simulink model "Level0"  (R2021a)
settings: Solver=VariableStepAuto  StartTime=0.0  StopTime=10.0  RelTol=1e-3
settings Model: Creator=jpss8  LastModifiedBy=jpss8

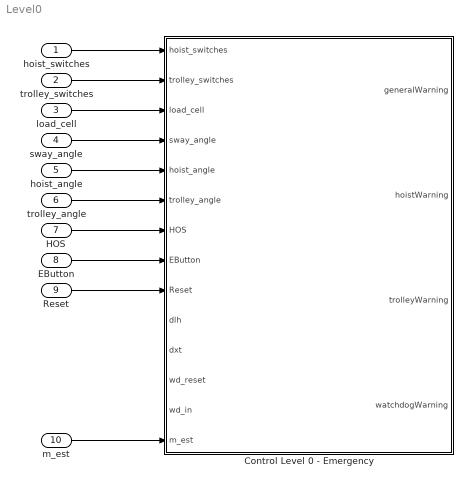
== system Level0 ==
  hoist_switches : Inport  PortDimensions=4
  trolley_switches : Inport  Port=2  PortDimensions=4
  load_cell : Inport  Port=3
  sway_angle : Inport  Port=4
  hoist_angle : Inport  Port=5
  trolley_angle : Inport  Port=6
  HOS : Inport  Port=7
  EButton : Inport  Port=8
  Reset : Inport  Port=9
  m_est : Inport  Port=10
  Control Level 0 - Emergency : Stateflow chart  TreatAsAtomicUnit=on
  wires:
  hoist_switches/1 -> Control Level 0 - Emergency/1(hoist_switches)
  trolley_switches/1 -> Control Level 0 - Emergency/2(trolley_switches)
  load_cell/1 -> Control Level 0 - Emergency/3(load_cell)
  sway_angle/1 -> Control Level 0 - Emergency/4(sway_angle)
  hoist_angle/1 -> Control Level 0 - Emergency/5(hoist_angle)
  trolley_angle/1 -> Control Level 0 - Emergency/6(trolley_angle)
  HOS/1 -> Control Level 0 - Emergency/7(HOS)
  EButton/1 -> Control Level 0 - Emergency/8(EButton)
  Reset/1 -> Control Level 0 - Emergency/9(Reset)
  m_est/1 -> Control Level 0 - Emergency/14(m_est)

== stateflow chart Level0/Control Level 0 - Emergency ==
  state Init
    generalWarning = 0;
    hoistWarning = 0;
    trolleyWarning = 0;
    watchdogWarning = 0;
  state Level0
    WD_TIMEOUT = 1000;
    state EMERGENCY [parallel]
      settings: executionOrder=2
      state NORMAL
        entry:
        generalWarning = 0;
        hoistWarning = 0;
        trolleyWarning = 0;
        during:
        VH_MAX = get_vh_max(m_est);
        VT_MAX = 3;
      state EMERGENCY_BUTTON
        entry:
        generalWarning = 1;
      state EMERGENCY_SWITCH_ACTIVATED
        state WAITING
        state TROLLEY_SWITCH
          entry:
          generalWarning = 0;
          trolleyWarning = 0;
        state HOIST_SWITCH
          entry:
          generalWarning = 0;
          hoistWarning = 0;
        (default) -> Level0.EMERGENCY.EMERGENCY_SWITCH_ACTIVATED.WAITING
        Level0.EMERGENCY.EMERGENCY_SWITCH_ACTIVATED.WAITING -> TROLLEY_SWITCH [order 1] : [check_trolley_switches(trolley_switches)]
        Level0.EMERGENCY.EMERGENCY_SWITCH_ACTIVATED.WAITING -> HOIST_SWITCH [order 2] : [check_hoist_switches(hoist_switches)]
      state SPEED_LIMIT
        during:
        state WAITING
        state SPEED_LIMIT_T
          entry:
          generalWarning = 0;
          trolleyWarning = 0;
        state SPEED_LIMIT_H
          entry:
          generalWarning = 0;
          hoistWarning = 0;
        (default) -> Level0.EMERGENCY.SPEED_LIMIT.WAITING
        Level0.EMERGENCY.SPEED_LIMIT.WAITING -> SPEED_LIMIT_H [order 1] : [dlh > VH_MAX]
        Level0.EMERGENCY.SPEED_LIMIT.WAITING -> SPEED_LIMIT_T [order 2] : [dxt > VT_MAX]
      state RESET_TO_NORMAL
        entry:
        generalWarning = 0;
        hoistWarning = 0;
        trolleyWarning = 0;
      state SAFETY
      (default) -> NORMAL
      RESET_TO_NORMAL -> NORMAL : [Reset]
      NORMAL -> EMERGENCY_BUTTON [order 3] : [EButton]
      NORMAL -> EMERGENCY_SWITCH_ACTIVATED [order 1] : [check_trolley_switches(trolley_switches) || check_hoist_switches(hoist_switches)]
      NORMAL -> SPEED_LIMIT [order 2] : [dxt > VT_MAX || dlh > VH_MAX]
      EMERGENCY_BUTTON -> RESET_TO_NORMAL : [Reset && ~EButton]
      SPEED_LIMIT -> SAFETY : [dxt < VT_MAX && dlh < VH_MAX]
      EMERGENCY_SWITCH_ACTIVATED -> SAFETY : [~check_hoist_switches(hoist_switches) && ~check_trolley_switches(trolley_switches) ]
      SAFETY -> RESET_TO_NORMAL : [Reset]
    state WATCHDOG [parallel]
      settings: executionOrder=1
      state Timer_Reset
        entry:
        wd_timer = 0;
        watchdogWarning = 0;
      state Falling_Edge
        during:
        wd_timer = wd_timer + 1
      state Rising_Edge
        during:
        wd_timer = wd_timer + 1
      state EMERGENCY
        % Emergency if timeout is reached
        watchdogWarning = 1;
      (default) -> Timer_Reset
      Level0.WATCHDOG.EMERGENCY -> Timer_Reset : [wd_reset == 1]
      Rising_Edge -> Timer_Reset [order 2] : [wd_in == 0]
      Timer_Reset -> Falling_Edge : [wd_in == 0]
      Falling_Edge -> Rising_Edge [order 1] : [wd_in == 1]
      Falling_Edge -> Level0.WATCHDOG.EMERGENCY [order 2] : [wd_timer > WD_TIMEOUT]
      Rising_Edge -> Level0.WATCHDOG.EMERGENCY [order 1] : [wd_timer > WD_TIMEOUT]
  (default) -> Init
  Init -> Level0
  data: switches function_input; hsw function_output; switches function_input; tsw function_output; ml function_input; vh_max function_output; hoist_switches input; trolley_switches input; load_cell input; sway_angle input; hoist_angle input; trolley_angle input; HOS input; EButton input; Reset input; wd_timer local; dlh input; dxt input; wd_reset input; wd_in input; WD_TIMEOUT local; VH_MAX local; m_est input; VT_MAX local; generalWarning output; hoistWarning output; trolleyWarning output; watchdogWarning output
  function hsw = check_trolley_switches(switches):
    | function hsw = check_trolley_switches(switches)
    | %{
    |     switches(1) -> Ship Side Switch
    |     switches(2) -> Ship Side Emergency Switch
    |     switches(3) -> Shore Side Switch
    |     switches(4) -> Shore Side Emergency Switch
    | %}
    |     if switches(2) || switches(4) % if any emergency switch is on then hsw = 1
    |         hsw = 1;
    |     else
    |         hsw = 0;
    |     end
    | end
  function tsw = check_hoist_switches(switches):
    | function tsw = check_hoist_switches(switches)
    | %{
    |     switches(1) -> Bottom Hoist Switch
    |     switches(2) -> Bottom Hoist Emergency Switch
    |     switches(3) -> Top Hoist Switch
    |     switches(4) -> Top Hoist Emergency Switch
    | %}
    |     if switches(2) || switches(4)
    |         tsw = 1;
    |     else
    |         tsw = 0;
    |     end
    | end
  function vh_max = get_vh_max(ml):
    | function vh_max = get_vh_max(ml)
    | 
    | % Max and minimum mass and speed values
    | min_m = 15000;
    | max_m = 65000;
    | min_v = 1.5;
    | max_v = 3;
    | 
    | P = max_m*min_v;  %65000 kg * 1.5 m/s
    | 
    | % Speed calculation at constant P
    | if (ml <= 32500)
    |     vh_max = max_v;
    | elseif (ml <= 65000)
    |     vh_max = P/ml;
    | else
    |     vh_max = 0;
    | end
    | 
    | end
